simulink model "ASM_Traffic_V2X_Complete_Model_2"  (R2019a)
settings: Solver=ode1  StartTime=SIM.tstart.v  StopTime=Inf  FixedStep=SIM.StepSize.v  RelTol=1e-3
PostLoadFcn:
  | if any(exist('dsrtsu_mdlpostloadfcn', 'file') ~= 0), dsrtsu_mdlpostloadfcn('Execute', bdroot); end
  | try, asm_mdl_postloadfcn(bdroot, 'UpdateModel', 2200); catch, disp(lasterr); end,
undefined symbols (not defined in the file): _SensorPnts_1, _SensorPnts_13, _SensorPnts_17, _SensorPnts_21, _SensorPnts_25, _SensorPnts_29, _SensorPnts_33, _SensorPnts_37, _SensorPnts_41, _SensorPnts_45, _SensorPnts_49, _SensorPnts_5, _SensorPnts_53, _SensorPnts_57, _SensorPnts_9, _to_, CPT, G5A, ITS, MDL, rad, s_to_rpm, SIM
libraries: simulink x169, ASM_VehicleDynamics_lib x126, ASM_Traffic_lib x83, ASM_Utils_lib x49, mdbs x45, ASM_Environment_lib x17, dspindex x12, dsaV2xLibraryAux x10, dsmpblib x6, dsaV2xAsn1Library x4, dsaV2xLibrary x4, ASM_BrakeHydraulics_lib x4
(part 10 of 36)

== system ASM_Traffic_V2X_Complete_Model_2/IO/V2X_Subsystem/Car_Data/Fellow_ID_3 ==
  "EGO_Car_Position " : Inport
  Input : Inport  Port=2
  Bus Creator : BusCreator  Inputs=6
  Bus Creator1 : BusCreator  Inputs=2
  Bus Selector1 : BusSelector  OutputSignals=Environment.Traffic.FellowMovement.FellowPositions.Pos_Fellows_MainPnt_CoorSys_E[x;y;z][m].Pos_x_Fellows[m],Environment.Traffic.FellowMovement.FellowPositions.Pos_Fellows_MainPnt_CoorSys_E[x;y;z][m].Pos_y_Fellows[m],Environment.Traffic.FellowMovement.FellowPositions.Pos_Fellows_MainPnt_CoorSys_E[x;y;z][m].Pos_z_Fellows[m],Environment.Traffic.FellowMovement.FellowVelocities.v_Fellows[x;y;z][km|h],Environment.Traffic.FellowMovement.FellowPositions.Angle_Fellows[x;y;z][deg].Angle_Yaw_Fellows[deg],Environment.Road.UserSignals_Customized.Const_Offset_Lat[deg],Environment.Road.UserSignals_Customized.Const_Offset_Long[deg]
  Display : Display
  Display1 : Display
  Distance_Calculation : Subsystem
  Fellow_ID : Constant  Value=3
  Fellow_ID_1_Spherical_XY2GPS : Subsystem  TreatAsAtomicUnit=on
  Heading Function : MATLAB Function  TreatAsAtomicUnit=on
  Terminator2 : Terminator
  Variable Selector{,1..3} (4 alike) : dspindex/Variable Selector  NumInputs=1  rowsOrCols=Rows  IdxMode=Variable  Elements=[1 3]  ZerOneIdxMode=One-based  errmode=Clip Index  FillMode=on  FillValues=0
  Output : Outport
  wires:
  Variable Selector3/1 -> Heading Function/1(u)  "Speed"
  Heading Function/1(y) -> Bus Creator/6  "Heading"
  Bus Selector1/5 -> Variable Selector3/1  "<Angle_Yaw_Fellows[deg]>"
  Variable Selector2/1 -> Bus Creator/5  "Speed"
  Bus Selector1/4 -> Variable Selector2/1  "<v_Fellows[x;y;z][km|h]>"
  Bus Selector1/1 -> Variable Selector/1  "<Pos_x_Fellows[m]>"
  Bus Selector1/3 -> Terminator2/1  "<Pos_z_Fellows[m]>"
  Bus Selector1/2 -> Variable Selector1/1  "<Pos_y_Fellows[m]>"
  Input/1 -> Bus Selector1/1
  Distance_Calculation/1(Distance<50m) -> Bus Creator/4  "Enable"
  "EGO_Car_Position "/1 -> Distance_Calculation/3(Egocar)
  Fellow_ID_1_Spherical_XY2GPS/2(Latitude_Veh) -> Bus Creator/2  "Latitude[deg]"
  Fellow_ID/1 -> Variable Selector/2, Variable Selector1/2, Variable Selector2/2, Variable Selector3/2, Bus Creator/3  "Fellow_ID"
  Variable Selector1/1 -> Display1/1, Distance_Calculation/1(Fellow_y), Fellow_ID_1_Spherical_XY2GPS/2(Position_y_Veh)
  Fellow_ID_1_Spherical_XY2GPS/1(Longitude_Veh) -> Bus Creator/1  "Longitude[deg]"
  Bus Creator/1 -> Output/1
  Variable Selector/1 -> Display/1, Distance_Calculation/2(Fellow_x), Fellow_ID_1_Spherical_XY2GPS/1(Position_x_Veh)
  Bus Selector1/6 -> Bus Creator1/1  "<Const_Offset_Lat[deg]>"
  Bus Selector1/7 -> Bus Creator1/2  "<Const_Offset_Long[deg]>"
  Bus Creator1/1 -> Fellow_ID_1_Spherical_XY2GPS/3(Lat_Long)

== system ASM_Traffic_V2X_Complete_Model_2/IO/V2X_Subsystem/Car_Data/Subsystem ==
  In1 : Inport
  Input : Inport  Port=2
  Input1 : Inport  Port=3
  Bus Creator : BusCreator  Inputs=5
  Bus Creator1 : BusCreator  Inputs=4
  Bus Selector : BusSelector  OutputSignals=Environment.Road.UserSignals_Customized.Const_Offset_Lat[deg],Environment.Road.UserSignals_Customized.Const_Offset_Long[deg],VehicleDynamics.VehicleMovement.Velocities.Vehicle.Linear.v_Total_Vehicle[km|h]
  Bus Selector1 : BusSelector  OutputSignals=Environment.Road.Road_ASMVeh.s_Veh_Road[m]
  Bus Selector2 : BusSelector  OutputSignals=Longitude[deg],Latitude[deg],Pos_y_Vehicle_CoorSys_E[m],Pos_x_Vehicle_CoorSys_E[m]
  Out1 : Outport
  wires:
  Bus Selector/2 -> Bus Creator1/2  "<Const_Offset_Long[deg]>"
  Bus Selector/1 -> Bus Creator1/1  "<Const_Offset_Lat[deg]>"
  In1/1 -> Bus Selector/1
  Input/1 -> Bus Selector2/1
  Bus Selector2/1 -> Bus Creator/1  "<Longitude[deg]>"
  Bus Selector2/2 -> Bus Creator/2  "<Latitude[deg]>"
  Bus Selector2/3 -> Bus Creator/3  "<Pos_y_Vehicle_CoorSys_E[m]>"
  Bus Creator/1 -> Bus Creator1/4
  Bus Creator1/1 -> Out1/1  "GenDENMData"
  Bus Selector2/4 -> Bus Creator/4  "<Pos_x_Vehicle_CoorSys_E[m]>"
  Bus Selector/3 -> Bus Creator1/3  "<v_Total_Vehicle[km|h]>"
  Input1/1 -> Bus Selector1/1
  Bus Selector1/1 -> Bus Creator/5  "<s_Veh_Road[m]>"

== system ASM_Traffic_V2X_Complete_Model_2/IO/V2X_Subsystem/Subsystem/Subsystem ==
  In1 : Inport
  Trigger : TriggerPort  VariantControl=Variant  PortDimensions=1
  Output : Outport
  wires:
  In1/1 -> Output/1

== system ASM_Traffic_V2X_Complete_Model_2/MDL/Drivetrain/External Loads/ManualLoadTorque ==
  In : Inport
  LoadTorque Switch : Switch  Criteria=u2 ~= 0  SaturateOnIntegerOverflow=on
  Sum : Sum  Inputs=|++  SaturateOnIntegerOverflow=on
  Out : Outport
  wires:
  [TAG_Drivetrain_SW_LoadTorque_Mode] -> LoadTorque Switch/2
  LoadTorque Switch/1 -> Out/1
  In/1 -> Sum/2, LoadTorque Switch/3
  [TAG_Drivetrain_Const_LoadTorque] -> Sum/1
  Sum/1 -> LoadTorque Switch/1

== system ASM_Traffic_V2X_Complete_Model_2/MDL/Drivetrain/Final_Drive_Assembly/ASMSignalCollector ==
  BusCreator : BusCreator  Inputs=13
  Clutch_4WD : Subsystem
  FinalDrive_Ratio : Subsystem
  Shaft_CF : Subsystem
  Shaft_CR : Subsystem
  Shaft_TGCL4WD : Subsystem
  Transfer_Gearbox : Subsystem
  tag scope: ASMBUS_Drivetrain_FinalDriveAssembly=global
  wires:
  [ASMBUS_Drivetrain_Clutch_4WD] -> Clutch_4WD/2(Clutch_4WD)
  [ASMBUS_Drivetrain_Transfer_Gearbox] -> Transfer_Gearbox/2(Transfer_Gearbox)
  [ASMBUS_Drivetrain_Shaft_CR] -> Shaft_CR/2(Shaft_CR)
  [ASMBUS_Drivetrain_Shaft_CF] -> Shaft_CF/2(Shaft_CF)
  [ASMBUS_Drivetrain_Shaft_TGCL4WD] -> Shaft_TGCL4WD/2(Shaft_TGCL4WD)
  [TAG_Sw_Drivetrain_Mode] -> Shaft_TGCL4WD/1(Drivetrain_Mode[1|2|3|4|5]), Shaft_CF/1(Drivetrain_Mode[1|2|3|4|5]), Shaft_CR/1(Drivetrain_Mode[1|2|3|4|5]), Transfer_Gearbox/1(Drivetrain_Mode[1|2|3|4|5]), Clutch_4WD/1(Drivetrain_Mode[1|2|3|4|5]), FinalDrive_Ratio/1(Drivetrain_Mode[1|2|3|4|5])
  FinalDrive_Ratio/1(i_FinalDrive[]) -> BusCreator/1
  Shaft_CR/1(ASMSignalBus) -> BusCreator/7
  Shaft_CF/1(ASMSignalBus) -> BusCreator/6
  BusCreator/1 -> [ASMBUS_Drivetrain_FinalDriveAssembly]  "FinalDriveAssembly"
  [ASMBUS_Drivetrain_FrontDifferential] -> BusCreator/3, FinalDrive_Ratio/3(FrontDifferential)
  [ASMBUS_Drivetrain_RearDifferential] -> BusCreator/4, FinalDrive_Ratio/4(RearDifferential)
  [ASMBUS_Drivetrain_Shaft_FL] -> BusCreator/10
  [ASMBUS_Drivetrain_Shaft_FR] -> BusCreator/11
  [ASMBUS_Drivetrain_Shaft_RL] -> BusCreator/12
  [ASMBUS_Drivetrain_Shaft_RR] -> BusCreator/13
  Shaft_TGCL4WD/1(ASMSignalBus) -> BusCreator/5
  [ASMBUS_Drivetrain_CentralDifferential] -> FinalDrive_Ratio/2(CentralDifferential), BusCreator/2
  Transfer_Gearbox/1(ASMSignalBus) -> BusCreator/8
  Clutch_4WD/1(ASMSignalBus) -> BusCreator/9

== system ASM_Traffic_V2X_Complete_Model_2/MDL/Drivetrain/Final_Drive_Assembly/Differentials ==
  Inertia_Trm[kgm2] : Inport
  Trq_Out_Trm[Nm] : Inport  Port=2
  Trq_In_FrontDiff[Nm] : Inport  Port=3
  Inertia_External_InputShaft_FrontDiff[kgm2] : Inport  Port=4
  Trq_Ext_Cage_FrontDiff[Nm] : Inport  Port=5
  Inertia_Ext_Cage_FrontDiff[kgm2] : Inport  Port=6
  Trq_In_RearDiff[Nm] : Inport  Port=7
  Inertia_External_InputShaft_RearDiff[kgm2] : Inport  Port=8
  Trq_RL_Shaft[Nm] : Inport  Port=9
  Trq_RR_Shaft[Nm] : Inport  Port=10
  Trq_CR_Shaft[Nm] : Inport  Port=11
  Trq_CF_Shaft[Nm] : Inport  Port=12
  Trq_FL_Shaft[Nm] : Inport  Port=13
  Trq_FR_Shaft[Nm] : Inport  Port=14
  Reset[0|1] : Inport  Port=15
  Bus Selector1 : BusSelector  OutputSignals=Ctrl_CentralDiff[%]
  Bus Selector2 : BusSelector  OutputSignals=Ctrl_Parking_Pawl[0|1]
  Bus Selector3 : BusSelector  OutputSignals=Ctrl_FrontDiff[%]
  Bus Selector4 : BusSelector  OutputSignals=Ctrl_RearDiff[%]
  CENTRAL_DIFFERENTIAL : ASM_VehicleDynamics_lib/Drivetrain/Differential/CENTRAL_DIFFERENTIAL  Tag=ASM_SUBCOMPONENT  Const_TrqDistribution=MDL.Drivetrain.CentralDifferential.Const_TrqDistribution  Const_i_MainReductionGear=MDL.Drivetrain.CentralDifferential.Const_i_MainReductionGear  Const_i_InnerGear=MDL.Drivetrain.CentralDifferential.Const_i_InnerGear  Const_Inertia_FrontSideGear=MDL.Drivetrain.CentralDifferential.Const_Inertia_FrontSideGear  Const_Inertia_RearSideGear=MDL.Drivetrain.CentralDifferential.Const_Inertia_RearSideGear  Const_Inertia_InnerGear=MDL.Drivetrain.CentralDifferential.Const_Inertia_InnerGear  Const_Inertia_MainReductionGear=MDL.Drivetrain.CentralDifferential.Const_Inertia_MainReductionGear  Const_Inertia_InputGear=MDL.Drivetrain.CentralDifferential.Const_Inertia_InputGear  Sw_DifferentialLock_Mode=MDL.Drivetrain.CentralDifferential.Sw_DifferentialLock_Mode  Const_Trq_Max_LockClutch=MDL.Drivetrain.CentralDifferential.Const_Trq_Max_LockClutch  Const_Coef_DynamicClutchTrq=MDL.Drivetrain.CentralDifferential.Const_Coef_DynamicClutchTrq  Const_Ctrl_Offset_LockClutch=MDL.Drivetrain.CentralDifferential.Const_Ctrl_Offset_LockClutch  StepSize=SIM.StepSize  ASMProperties=struct('Name','CENTRAL_DIFFERENTIAL','Version','8.0','Library','ASM_VehicleDynamics_lib')  ASMInstanceName=central_differential  ASMInstanceID=1
  Ctrl_Parking_Pawl_FrontDiff[0|1] : Constant  Value=0
  Ctrl_Parking_Pawl_RearDiff[0|1] : Constant  Value=0
  FROM_STABILIZATION_CENTRAL_DIFFERENTIAL : ASM_VehicleDynamics_lib/Drivetrain/Stabilization/FROM_STABILIZATION  Tag=ASM_SUBCOMPONENT  Stabi_Block=CENTRAL_DIFFERENTIAL  Stabi_Block_ID=1  ASMProperties=struct('Name','FROM_STABILIZATION','Version','1.0','Library','ASM_VehicleDynamics_lib')  ASMInstanceName=from_stabilization  ASMInstanceID=1
      settings: AttributesFormatString=Destination: CENTRAL_DIFFERENTIAL_ID1
  FROM_STABILIZATION_FRONT_DIFFERENTIAL : ASM_VehicleDynamics_lib/Drivetrain/Stabilization/FROM_STABILIZATION  Tag=ASM_SUBCOMPONENT  Stabi_Block=FRONT_DIFFERENTIAL  Stabi_Block_ID=1  ASMProperties=struct('Name','FROM_STABILIZATION','Version','1.0','Library','ASM_VehicleDynamics_lib')  ASMInstanceName=from_stabilization  ASMInstanceID=1
      settings: AttributesFormatString=Destination: FRONT_DIFFERENTIAL_ID1
  FROM_STABILIZATION_REAR_DIFFERENTIAL : ASM_VehicleDynamics_lib/Drivetrain/Stabilization/FROM_STABILIZATION  Tag=ASM_SUBCOMPONENT  Stabi_Block=REAR_DIFFERENTIAL  Stabi_Block_ID=1  ASMProperties=struct('Name','FROM_STABILIZATION','Version','1.0','Library','ASM_VehicleDynamics_lib')  ASMInstanceName=from_stabilization  ASMInstanceID=1
      settings: AttributesFormatString=Destination: REAR_DIFFERENTIAL_ID1
  FRONT_DIFFERENTIAL : ASM_VehicleDynamics_lib/Drivetrain/Differential/FRONT_DIFFERENTIAL  Tag=ASM_SUBCOMPONENT  Const_i_MainReductionGear=MDL.Drivetrain.FrontDifferential.Const_i_MainReductionGear  Const_i_InnerGear=MDL.Drivetrain.FrontDifferential.Const_i_InnerGear  Const_Inertia_LeftSideGear=MDL.Drivetrain.FrontDifferential.Const_Inertia_LeftSideGear  Const_Inertia_RightSideGear=MDL.Drivetrain.FrontDifferential.Const_Inertia_RightSideGear  Const_Inertia_InnerGear=MDL.Drivetrain.FrontDifferential.Const_Inertia_InnerGear  Const_Inertia_MainReductionGear=MDL.Drivetrain.FrontDifferential.Const_Inertia_MainReductionGear  Const_Inertia_InputGear=MDL.Drivetrain.FrontDifferential.Const_Inertia_InputGear  Sw_DifferentialLock_Mode=MDL.Drivetrain.FrontDifferential.Sw_DifferentialLock_Mode  Const_Trq_Max_LockClutch=MDL.Drivetrain.FrontDifferential.Const_Trq_Max_LockClutch  Const_Coef_DynamicClutchTrq=MDL.Drivetrain.FrontDifferential.Const_Coef_DynamicClutchTrq  Const_Ctrl_Offset_LockClutch=MDL.Drivetrain.FrontDifferential.Const_Ctrl_Offset_LockClutch  StepSize=SIM.StepSize  ASMProperties=struct('Name','FRONT_DIFFERENTIAL','Version','8.0','Library','ASM_VehicleDynamics_lib')  ASMInstanceName=front_differential  ASMInstanceID=1
  Inertia_Ext_Cage_CentralDiff[kgm2] : Constant  Value=0
  Inertia_Ext_Cage_RearDiff[kgm2] : Constant  Value=0
  REAR_DIFFERENTIAL : ASM_VehicleDynamics_lib/Drivetrain/Differential/REAR_DIFFERENTIAL  Tag=ASM_SUBCOMPONENT  Const_i_MainReductionGear=MDL.Drivetrain.RearDifferential.Const_i_MainReductionGear  Const_i_InnerGear=MDL.Drivetrain.RearDifferential.Const_i_InnerGear  Const_Inertia_LeftSideGear=MDL.Drivetrain.RearDifferential.Const_Inertia_LeftSideGear  Const_Inertia_RightSideGear=MDL.Drivetrain.RearDifferential.Const_Inertia_RightSideGear  Const_Inertia_InnerGear=MDL.Drivetrain.RearDifferential.Const_Inertia_InnerGear  Const_Inertia_MainReductionGear=MDL.Drivetrain.RearDifferential.Const_Inertia_MainReductionGear  Const_Inertia_InputGear=MDL.Drivetrain.RearDifferential.Const_Inertia_InputGear  Sw_DifferentialLock_Mode=MDL.Drivetrain.RearDifferential.Sw_DifferentialLock_Mode  Const_Trq_Max_LockClutch=MDL.Drivetrain.RearDifferential.Const_Trq_Max_LockClutch  Const_Coef_DynamicClutchTrq=MDL.Drivetrain.RearDifferential.Const_Coef_DynamicClutchTrq  Const_Ctrl_Offset_LockClutch=MDL.Drivetrain.RearDifferential.Const_Ctrl_Offset_LockClutch  StepSize=SIM.StepSize  ASMProperties=struct('Name','REAR_DIFFERENTIAL','Version','8.0','Library','ASM_VehicleDynamics_lib')  ASMInstanceName=rear_differential  ASMInstanceID=1
  Saturation[1_3] : Saturate  UpperLimit=3  LowerLimit=1
  SignalSelection : Subsystem
  TO_STABILIZATION_CENTRAL_DIFFERENTIAL : ASM_VehicleDynamics_lib/Drivetrain/Stabilization/TO_STABILIZATION  Tag=ASM_SUBCOMPONENT  Stabi_Block=CENTRAL_DIFFERENTIAL  Stabi_Block_ID=1  ASMProperties=struct('Name','TO_STABILIZATION','Version','1.0','Library','ASM_VehicleDynamics_lib')  ASMInstanceName=to_stabilization  ASMInstanceID=1
      settings: AttributesFormatString=Source: CENTRAL_DIFFERENTIAL_ID1
  TO_STABILIZATION_FRONT_DIFFERENTIAL : ASM_VehicleDynamics_lib/Drivetrain/Stabilization/TO_STABILIZATION  Tag=ASM_SUBCOMPONENT  Stabi_Block=FRONT_DIFFERENTIAL  Stabi_Block_ID=1  ASMProperties=struct('Name','TO_STABILIZATION','Version','1.0','Library','ASM_VehicleDynamics_lib')  ASMInstanceName=to_stabilization  ASMInstanceID=1
      settings: AttributesFormatString=Source: FRONT_DIFFERENTIAL_ID1
  TO_STABILIZATION_REAR_DIFFERENTIAL : ASM_VehicleDynamics_lib/Drivetrain/Stabilization/TO_STABILIZATION  Tag=ASM_SUBCOMPONENT  Stabi_Block=REAR_DIFFERENTIAL  Stabi_Block_ID=1  ASMProperties=struct('Name','TO_STABILIZATION','Version','1.0','Library','ASM_VehicleDynamics_lib')  ASMInstanceName=to_stabilization  ASMInstanceID=1
      settings: AttributesFormatString=Source: REAR_DIFFERENTIAL_ID1
  Trq_Ext_Cage_CentralDiff[Nm] : Constant  Value=0
  Trq_Ext_Cage_RearDiff[Nm] : Constant  Value=0
  omega_Cage_CentralDiff[rad|s] : Terminator
  omega_Cage_RearDiff[rad|s] : Terminator
  omega_Out_Front_Init_CentralDiff[rad|s] : Constant  Value=0
  omega_Out_Left_Init_FrontDiff[rad|s] : Constant  Value=0
  omega_Out_Left_Init_RearDiff[rad|s] : Constant  Value=0
  omega_Out_Rear_Init_CentralDiff[rad|s] : Constant  Value=0
  omega_Out_Right_Init_FrontDiff[rad|s] : Constant  Value=0
  omega_Out_Right_Init_RearDiff[rad|s] : Constant  Value=0
  omega_In_Diff[rad|s] : Outport
  omega_Cage_FrontDiff[rad|s] : Outport  Port=2
  omega_In_RearDiff[rad|s] : Outport  Port=3
  omega_In_FrontDiff[rad|s] : Outport  Port=4
  omega_Out_Front_CentralDiff[rad|s] : Outport  Port=5
  omega_Out_Rear_CentralDiff[rad|s] : Outport  Port=6
  omega_Out_Left_FrontDiff[rad|s] : Outport  Port=7
  omega_Out_Right_FrontDiff[rad|s] : Outport  Port=8
  omega_Out_Left_RearDiff[rad|s] : Outport  Port=9
  omega_Out_Right_RearDiff[rad|s] : Outport  Port=10
  tag scope: ASMBUS_Drivetrain_CentralDifferential=scoped, ASMBUS_Drivetrain_FrontDifferential=scoped, ASMBUS_Drivetrain_RearDifferential=scoped
  wires:
  omega_Out_Right_Init_RearDiff[rad|s]/1 -> REAR_DIFFERENTIAL/11
  Trq_Ext_Cage_RearDiff[Nm]/1 -> REAR_DIFFERENTIAL/7
  omega_Out_Left_Init_RearDiff[rad|s]/1 -> REAR_DIFFERENTIAL/10
  Inertia_Ext_Cage_RearDiff[kgm2]/1 -> REAR_DIFFERENTIAL/8
  Ctrl_Parking_Pawl_RearDiff[0|1]/1 -> REAR_DIFFERENTIAL/9
  REAR_DIFFERENTIAL/5 -> omega_Cage_RearDiff[rad|s]/1
  omega_Out_Right_Init_FrontDiff[rad|s]/1 -> FRONT_DIFFERENTIAL/11
  omega_Out_Left_Init_FrontDiff[rad|s]/1 -> FRONT_DIFFERENTIAL/10
  Ctrl_Parking_Pawl_FrontDiff[0|1]/1 -> FRONT_DIFFERENTIAL/9
  FRONT_DIFFERENTIAL/1 -> [ASMBUS_Drivetrain_FrontDifferential]
  Inertia_Ext_Cage_CentralDiff[kgm2]/1 -> CENTRAL_DIFFERENTIAL/10
  Trq_Ext_Cage_CentralDiff[Nm]/1 -> CENTRAL_DIFFERENTIAL/9
  omega_Out_Front_Init_CentralDiff[rad|s]/1 -> CENTRAL_DIFFERENTIAL/11
  omega_Out_Rear_Init_CentralDiff[rad|s]/1 -> CENTRAL_DIFFERENTIAL/12
  CENTRAL_DIFFERENTIAL/5 -> omega_Cage_CentralDiff[rad|s]/1
  CENTRAL_DIFFERENTIAL/4 -> omega_Out_Rear_CentralDiff[rad|s]/1
  CENTRAL_DIFFERENTIAL/3 -> omega_Out_Front_CentralDiff[rad|s]/1
  CENTRAL_DIFFERENTIAL/2 -> SignalSelection/1(omega_In_CentralDiff[rad|s])
  CENTRAL_DIFFERENTIAL/1 -> [ASMBUS_Drivetrain_CentralDifferential]
  Reset[0|1]/1 -> CENTRAL_DIFFERENTIAL/7, REAR_DIFFERENTIAL/5, FRONT_DIFFERENTIAL/5
  Saturation[1_3]/1 -> CENTRAL_DIFFERENTIAL/4
  [TAG_Sw_Drivetrain_Mode] -> Saturation[1_3]/1
  SignalSelection/1(omega_In_Diff[rad|s]) -> omega_In_Diff[rad|s]/1
  Inertia_Ext_Cage_FrontDiff[kgm2]/1 -> FRONT_DIFFERENTIAL/8
  Trq_Ext_Cage_FrontDiff[Nm]/1 -> FRONT_DIFFERENTIAL/7
  Trq_In_RearDiff[Nm]/1 -> REAR_DIFFERENTIAL/1
  Trq_CF_Shaft[Nm]/1 -> CENTRAL_DIFFERENTIAL/6
  REAR_DIFFERENTIAL/2 -> omega_In_RearDiff[rad|s]/1
  FRONT_DIFFERENTIAL/2 -> SignalSelection/2(omega_In_FrontDiff[rad|s]), omega_In_FrontDiff[rad|s]/1
  [TAG_FromIO_Drivetrain] -> Bus Selector1/1, Bus Selector2/1, Bus Selector3/1, Bus Selector4/1
  Trq_In_FrontDiff[Nm]/1 -> FRONT_DIFFERENTIAL/1
  Bus Selector1/1 -> CENTRAL_DIFFERENTIAL/3  "<Ctrl_CentralDiff[%]>"
  Bus Selector3/1 -> FRONT_DIFFERENTIAL/2  "<Ctrl_FrontDiff[%]>"
  Trq_CR_Shaft[Nm]/1 -> CENTRAL_DIFFERENTIAL/5
  FRONT_DIFFERENTIAL/5 -> omega_Cage_FrontDiff[rad|s]/1
  Inertia_External_InputShaft_FrontDiff[kgm2]/1 -> FRONT_DIFFERENTIAL/6
  Bus Selector4/1 -> REAR_DIFFERENTIAL/2  "<Ctrl_RearDiff[%]>"
  Inertia_Trm[kgm2]/1 -> CENTRAL_DIFFERENTIAL/1
  Trq_Out_Trm[Nm]/1 -> CENTRAL_DIFFERENTIAL/2
  REAR_DIFFERENTIAL/1 -> [ASMBUS_Drivetrain_RearDifferential]
  Inertia_External_InputShaft_RearDiff[kgm2]/1 -> REAR_DIFFERENTIAL/6
  Bus Selector2/1 -> CENTRAL_DIFFERENTIAL/8  "<Ctrl_Parking_Pawl[0|1]>"
  Trq_RL_Shaft[Nm]/1 -> REAR_DIFFERENTIAL/3
  Trq_RR_Shaft[Nm]/1 -> REAR_DIFFERENTIAL/4
  REAR_DIFFERENTIAL/3 -> omega_Out_Left_RearDiff[rad|s]/1
  Trq_FR_Shaft[Nm]/1 -> FRONT_DIFFERENTIAL/4
  REAR_DIFFERENTIAL/4 -> omega_Out_Right_RearDiff[rad|s]/1
  FRONT_DIFFERENTIAL/3 -> omega_Out_Left_FrontDiff[rad|s]/1
  FRONT_DIFFERENTIAL/4 -> omega_Out_Right_FrontDiff[rad|s]/1
  Trq_FL_Shaft[Nm]/1 -> FRONT_DIFFERENTIAL/3
  FRONT_DIFFERENTIAL/6 -> TO_STABILIZATION_FRONT_DIFFERENTIAL/1
  REAR_DIFFERENTIAL/6 -> TO_STABILIZATION_REAR_DIFFERENTIAL/1
  FROM_STABILIZATION_REAR_DIFFERENTIAL/1 -> REAR_DIFFERENTIAL/12
  FROM_STABILIZATION_FRONT_DIFFERENTIAL/1 -> FRONT_DIFFERENTIAL/12
  CENTRAL_DIFFERENTIAL/6 -> TO_STABILIZATION_CENTRAL_DIFFERENTIAL/1
  FROM_STABILIZATION_CENTRAL_DIFFERENTIAL/1 -> CENTRAL_DIFFERENTIAL/13

== system ASM_Traffic_V2X_Complete_Model_2/MDL/Drivetrain/Final_Drive_Assembly/FF4WD_Parts ==
  Trq_RL_Shaft[Nm] : Inport
  Trq_RR_Shaft[Nm] : Inport  Port=2
  Reset[0|1] : Inport  Port=3
  omega_In_RearDiff[rad|s] : Inport  Port=4
  omega_Cage_FrontDiff[rad|s] : Inport  Port=5
  Bus Selector1 : BusSelector  OutputSignals=Const_i_MainReductionGear[]
  Bus Selector4 : BusSelector  OutputSignals=Ctrl_Clutch_4WD[%]
  CLUTCH_4WD : ASM_VehicleDynamics_lib/Drivetrain/Clutch/CLUTCH_4WD  Tag=ASM_SUBCOMPONENT  Const_Inertia_InputSide=MDL.Drivetrain.Clutch_4WD.Const_Inertia_InputSide  Const_Inertia_OutputSide=MDL.Drivetrain.Clutch_4WD.Const_Inertia_OutputSide  Const_Torque_Max=MDL.Drivetrain.Clutch_4WD.Const_Torque_Max  Map_Trq_Clutch_Red=MDL.Drivetrain.Clutch_4WD.Map_Trq_Clutch_Red  Const_Coef_DynamicClutchTrq=MDL.Drivetrain.Clutch_4WD.Const_Coef_DynamicClutchTrq  StepSize=SIM.StepSize  ASMProperties=struct('Name','CLUTCH_4WD','Version','6.0','Library','ASM_VehicleDynamics_lib')  ASMInstanceName=clutch_4wd  ASMInstanceID=1
  FROM_STABILIZATION_CLUTCH_4WD : ASM_VehicleDynamics_lib/Drivetrain/Stabilization/FROM_STABILIZATION  Tag=ASM_SUBCOMPONENT  Stabi_Block=CLUTCH_4WD  Stabi_Block_ID=1  ASMProperties=struct('Name','FROM_STABILIZATION','Version','1.0','Library','ASM_VehicleDynamics_lib')  ASMInstanceName=from_stabilization  ASMInstanceID=1
      settings: AttributesFormatString=Destination: CLUTCH_4WD_ID1
  Map_Mode_2_Parameter : Lookup_n-D  NumberOfTableDimensions=1  BreakpointsForDimension1=[1:5]  Table=[1 2 3 1 2]  InternalRulePriority=Speed  RndMeth=Simplest  InputSameDT=on
      settings: AttributesFormatString=Map FF => FWD & FF4WD => AWD
  SHAFT_TGCL4WD : ASM_VehicleDynamics_lib/Drivetrain/Shaft/SHAFT_TGCL4WD  Tag=ASM_SUBCOMPONENT  Const_Stiffness_Shaft_TGCL4WD=MDL.Drivetrain.Shaft_TGCL4WD.Const_Stiffness  Const_Damping_Shaft_TGCL4WD=MDL.Drivetrain.Shaft_TGCL4WD.Const_Damping  StepSize=SIM.StepSize  ASMProperties=struct('Name','SHAFT_TGCL4WD','Version','4.0','Library','ASM_VehicleDynamics_lib')  ASMInstanceName=Shafts  ASMInstanceID=1
  TO_STABILIZATION_CLUTCH_4WD : ASM_VehicleDynamics_lib/Drivetrain/Stabilization/TO_STABILIZATION  Tag=ASM_SUBCOMPONENT  Stabi_Block=CLUTCH_4WD  Stabi_Block_ID=1  ASMProperties=struct('Name','TO_STABILIZATION','Version','1.0','Library','ASM_VehicleDynamics_lib')  ASMInstanceName=to_stabilization  ASMInstanceID=1
      settings: AttributesFormatString=Source: CLUTCH_4WD_ID1
  TO_STABILIZATION_SHAFT_TGCL4WD : ASM_VehicleDynamics_lib/Drivetrain/Stabilization/TO_STABILIZATION  Tag=ASM_SUBCOMPONENT  Stabi_Block=SHAFT_TGCL4WD  Stabi_Block_ID=1  ASMProperties=struct('Name','TO_STABILIZATION','Version','1.0','Library','ASM_VehicleDynamics_lib')  ASMInstanceName=to_stabilization  ASMInstanceID=1
      settings: AttributesFormatString=Source: SHAFT_TGCL4WD_ID1
  TO_STABILIZATION_TRANSFER_GEARBOX : ASM_VehicleDynamics_lib/Drivetrain/Stabilization/TO_STABILIZATION  Tag=ASM_SUBCOMPONENT  Stabi_Block=TRANSFER_GEARBOX  Stabi_Block_ID=1  ASMProperties=struct('Name','TO_STABILIZATION','Version','1.0','Library','ASM_VehicleDynamics_lib')  ASMInstanceName=to_stabilization  ASMInstanceID=1
      settings: AttributesFormatString=Source: TRANSFER_GEARBOX_ID1
  TRANSFER_GEARBOX : ASM_VehicleDynamics_lib/Drivetrain/Gearbox/TRANSFER_GEARBOX  Tag=ASM_SUBCOMPONENT  Const_GearRatio=MDL.Drivetrain.TransferGearbox.Const_GearRatio  Const_Inertia_Output_Gear=MDL.Drivetrain.TransferGearbox.Const_Inertia_Output_Gear  Const_Inertia_Input_Gear=MDL.Drivetrain.TransferGearbox.Const_Inertia_Input_Gear  ASMProperties=struct('Name','TRANSFER_GEARBOX','Version','4.0','Library','ASM_VehicleDynamics_lib')  ASMInstanceName=transfer_gearbox  ASMInstanceID=1
  omega_Clutch_4WD_In_Init[rad|s] : Constant  Value=0
  Inertia_Out_Clutch4WD[kgm2] : Outport
  Trq_Lock_Clutch4WD[Nm] : Outport  Port=2
  Inertia_In_TransferGearbox[kgm2] : Outport  Port=3
  Trq_In_TransferGearbox[Nm] : Outport  Port=4
  tag scope: ASMBUS_Drivetrain_Clutch_4WD=scoped, ASMBUS_Drivetrain_Shaft_TGCL4WD=scoped, ASMBUS_Drivetrain_Transfer_Gearbox=scoped
  wires:
  omega_Cage_FrontDiff[rad|s]/1 -> TRANSFER_GEARBOX/3
  omega_Clutch_4WD_In_Init[rad|s]/1 -> CLUTCH_4WD/8
  Bus Selector1/1 -> CLUTCH_4WD/7  "<Const_i_MainReductionGear[]>"
  [ASMBUS_Drivetrain_RearDifferential] -> Bus Selector1/1
  TRANSFER_GEARBOX/3 -> Inertia_In_TransferGearbox[kgm2]/1
  TRANSFER_GEARBOX/2 -> Trq_In_TransferGearbox[Nm]/1
  TRANSFER_GEARBOX/1 -> [ASMBUS_Drivetrain_Transfer_Gearbox]
  CLUTCH_4WD/4 -> Inertia_Out_Clutch4WD[kgm2]/1
  CLUTCH_4WD/3 -> Trq_Lock_Clutch4WD[Nm]/1
  SHAFT_TGCL4WD/1 -> [ASMBUS_Drivetrain_Shaft_TGCL4WD]
  [TAG_FromIO_Drivetrain] -> Bus Selector4/1
  Bus Selector4/1 -> CLUTCH_4WD/2  "<Ctrl_Clutch_4WD[%]>"
  [TAG_Sw_Drivetrain_Mode] -> Map_Mode_2_Parameter/1
  Map_Mode_2_Parameter/1 -> SHAFT_TGCL4WD/3, TRANSFER_GEARBOX/1
  Reset[0|1]/1 -> CLUTCH_4WD/6, SHAFT_TGCL4WD/4
  omega_In_RearDiff[rad|s]/1 -> CLUTCH_4WD/5
  Trq_RR_Shaft[Nm]/1 -> CLUTCH_4WD/4
  Trq_RL_Shaft[Nm]/1 -> CLUTCH_4WD/3
  CLUTCH_4WD/2 -> SHAFT_TGCL4WD/2
  TRANSFER_GEARBOX/4 -> SHAFT_TGCL4WD/1
  SHAFT_TGCL4WD/2 -> CLUTCH_4WD/1, TRANSFER_GEARBOX/2
  CLUTCH_4WD/1 -> [ASMBUS_Drivetrain_Clutch_4WD]
  TRANSFER_GEARBOX/5 -> TO_STABILIZATION_TRANSFER_GEARBOX/1
  SHAFT_TGCL4WD/3 -> TO_STABILIZATION_SHAFT_TGCL4WD/1
  CLUTCH_4WD/5 -> TO_STABILIZATION_CLUTCH_4WD/1
  FROM_STABILIZATION_CLUTCH_4WD/1 -> CLUTCH_4WD/9

== system ASM_Traffic_V2X_Complete_Model_2/MDL/Drivetrain/Final_Drive_Assembly/STABILIZATION ==
  DRIVETRAIN_STABILIZATION : ASM_VehicleDynamics_lib/Drivetrain/Stabilization/DRIVETRAIN_STABILIZATION  Tag=ASM_SUBCOMPONENT  StepSize=SIM.StepSize  ASMProperties=struct('Name','DRIVETRAIN_STABILIZATION','Version','1.0','Library','ASM_VehicleDynamics_lib')  ASMInstanceName=drivetrain_stabilization  ASMInstanceID=1
  FROM_ASM_CENTRAL_DIFFERENTIAL : ASM_VehicleDynamics_lib/Drivetrain/Stabilization/FROM_ASM  Tag=ASM_SUBCOMPONENT  Stabi_Block=CENTRAL_DIFFERENTIAL  Stabi_Block_ID=1  ASMProperties=struct('Name','FROM_ASM','Version','1.0','Library','ASM_VehicleDynamics_lib')  ASMInstanceName=from_asm  ASMInstanceID=1
      settings: AttributesFormatString=Source: CENTRAL_DIFFERENTIAL_ID1
  FROM_ASM_CLUTCH : ASM_VehicleDynamics_lib/Drivetrain/Stabilization/FROM_ASM  Tag=ASM_SUBCOMPONENT  Stabi_Block=CLUTCH  Stabi_Block_ID=1  ASMProperties=struct('Name','FROM_ASM','Version','1.0','Library','ASM_VehicleDynamics_lib')  ASMInstanceName=from_asm  ASMInstanceID=1
      settings: AttributesFormatString=Source: CLUTCH_ID1
  FROM_ASM_CLUTCH_4WD : ASM_VehicleDynamics_lib/Drivetrain/Stabilization/FROM_ASM  Tag=ASM_SUBCOMPONENT  Stabi_Block=CLUTCH_4WD  Stabi_Block_ID=1  ASMProperties=struct('Name','FROM_ASM','Version','1.0','Library','ASM_VehicleDynamics_lib')  ASMInstanceName=from_asm  ASMInstanceID=1
      settings: AttributesFormatString=Source: CLUTCH_4WD_ID1
  FROM_ASM_CRANK_SHAFT : ASM_VehicleDynamics_lib/Drivetrain/Stabilization/FROM_ASM  Tag=ASM_SUBCOMPONENT  Stabi_Block=CRANK_SHAFT  Stabi_Block_ID=1  ASMProperties=struct('Name','FROM_ASM','Version','1.0','Library','ASM_VehicleDynamics_lib')  ASMInstanceName=from_asm  ASMInstanceID=1
      settings: AttributesFormatString=Source: CRANK_SHAFT_ID1
  FROM_ASM_FRONT_DIFFERENTIAL : ASM_VehicleDynamics_lib/Drivetrain/Stabilization/FROM_ASM  Tag=ASM_SUBCOMPONENT  Stabi_Block=FRONT_DIFFERENTIAL  Stabi_Block_ID=1  ASMProperties=struct('Name','FROM_ASM','Version','1.0','Library','ASM_VehicleDynamics_lib')  ASMInstanceName=from_asm  ASMInstanceID=1
      settings: AttributesFormatString=Source: FRONT_DIFFERENTIAL_ID1
  FROM_ASM_GEARBOX : ASM_VehicleDynamics_lib/Drivetrain/Stabilization/FROM_ASM  Tag=ASM_SUBCOMPONENT  Stabi_Block=GEARBOX  Stabi_Block_ID=1  ASMProperties=struct('Name','FROM_ASM','Version','1.0','Library','ASM_VehicleDynamics_lib')  ASMInstanceName=from_asm  ASMInstanceID=1
      settings: AttributesFormatString=Source: GEARBOX_ID1
  FROM_ASM_REAR_DIFFERENTIAL : ASM_VehicleDynamics_lib/Drivetrain/Stabilization/FROM_ASM  Tag=ASM_SUBCOMPONENT  Stabi_Block=REAR_DIFFERENTIAL  Stabi_Block_ID=1  ASMProperties=struct('Name','FROM_ASM','Version','1.0','Library','ASM_VehicleDynamics_lib')  ASMInstanceName=from_asm  ASMInstanceID=1
      settings: AttributesFormatString=Source: REAR_DIFFERENTIAL_ID1
  FROM_ASM_SHAFT_CF : ASM_VehicleDynamics_lib/Drivetrain/Stabilization/FROM_ASM  Tag=ASM_SUBCOMPONENT  Stabi_Block=SHAFT_CF  Stabi_Block_ID=1  ASMProperties=struct('Name','FROM_ASM','Version','1.0','Library','ASM_VehicleDynamics_lib')  ASMInstanceName=from_asm  ASMInstanceID=1
      settings: AttributesFormatString=Source: SHAFT_CF_ID1
  FROM_ASM_SHAFT_CR : ASM_VehicleDynamics_lib/Drivetrain/Stabilization/FROM_ASM  Tag=ASM_SUBCOMPONENT  Stabi_Block=SHAFT_CR  Stabi_Block_ID=1  ASMProperties=struct('Name','FROM_ASM','Version','1.0','Library','ASM_VehicleDynamics_lib')  ASMInstanceName=from_asm  ASMInstanceID=1
      settings: AttributesFormatString=Source: SHAFT_CR_ID1
  FROM_ASM_SHAFT_FL : ASM_VehicleDynamics_lib/Drivetrain/Stabilization/FROM_ASM  Tag=ASM_SUBCOMPONENT  Stabi_Block=SHAFT_FL  Stabi_Block_ID=1  ASMProperties=struct('Name','FROM_ASM','Version','1.0','Library','ASM_VehicleDynamics_lib')  ASMInstanceName=from_asm  ASMInstanceID=1
      settings: AttributesFormatString=Source: SHAFT_FL_ID1
  FROM_ASM_SHAFT_FR : ASM_VehicleDynamics_lib/Drivetrain/Stabilization/FROM_ASM  Tag=ASM_SUBCOMPONENT  Stabi_Block=SHAFT_FR  Stabi_Block_ID=1  ASMProperties=struct('Name','FROM_ASM','Version','1.0','Library','ASM_VehicleDynamics_lib')  ASMInstanceName=from_asm  ASMInstanceID=1
      settings: AttributesFormatString=Source: SHAFT_FR_ID1
  FROM_ASM_SHAFT_RL : ASM_VehicleDynamics_lib/Drivetrain/Stabilization/FROM_ASM  Tag=ASM_SUBCOMPONENT  Stabi_Block=SHAFT_RL  Stabi_Block_ID=1  ASMProperties=struct('Name','FROM_ASM','Version','1.0','Library','ASM_VehicleDynamics_lib')  ASMInstanceName=from_asm  ASMInstanceID=1
      settings: AttributesFormatString=Source: SHAFT_RL_ID1
  FROM_ASM_SHAFT_RR : ASM_VehicleDynamics_lib/Drivetrain/Stabilization/FROM_ASM  Tag=ASM_SUBCOMPONENT  Stabi_Block=SHAFT_RR  Stabi_Block_ID=1  ASMProperties=struct('Name','FROM_ASM','Version','1.0','Library','ASM_VehicleDynamics_lib')  ASMInstanceName=from_asm  ASMInstanceID=1
      settings: AttributesFormatString=Source: SHAFT_RR_ID1
  FROM_ASM_SHAFT_TGCL4WD : ASM_VehicleDynamics_lib/Drivetrain/Stabilization/FROM_ASM  Tag=ASM_SUBCOMPONENT  Stabi_Block=SHAFT_TGCL4WD  Stabi_Block_ID=1  ASMProperties=struct('Name','FROM_ASM','Version','1.0','Library','ASM_VehicleDynamics_lib')  ASMInstanceName=from_asm  ASMInstanceID=1
      settings: AttributesFormatString=Source: SHAFT_TGCL4WD_ID1
  FROM_ASM_TORQUE_CONVERTER : ASM_VehicleDynamics_lib/Drivetrain/Stabilization/FROM_ASM  Tag=ASM_SUBCOMPONENT  Stabi_Block=TORQUE_CONVERTER  Stabi_Block_ID=1  ASMProperties=struct('Name','FROM_ASM','Version','1.0','Library','ASM_VehicleDynamics_lib')  ASMInstanceName=from_asm  ASMInstanceID=1
      settings: AttributesFormatString=Source: TORQUE_CONVERTER_ID1
  FROM_ASM_TRANSFER_GEARBOX : ASM_VehicleDynamics_lib/Drivetrain/Stabilization/FROM_ASM  Tag=ASM_SUBCOMPONENT  Stabi_Block=TRANSFER_GEARBOX  Stabi_Block_ID=1  ASMProperties=struct('Name','FROM_ASM','Version','1.0','Library','ASM_VehicleDynamics_lib')  ASMInstanceName=from_asm  ASMInstanceID=1
      settings: AttributesFormatString=Source: TRANSFER_GEARBOX_ID1
  Saturation[1_5] : Saturate  UpperLimit=5  LowerLimit=1
  TO_ASM_CENTRAL_DIFFERENTIAL : ASM_VehicleDynamics_lib/Drivetrain/Stabilization/TO_ASM  Tag=ASM_SUBCOMPONENT  Stabi_Block=CENTRAL_DIFFERENTIAL  Stabi_Block_ID=1  ASMProperties=struct('Name','TO_ASM','Version','1.0','Library','ASM_VehicleDynamics_lib')  ASMInstanceName=to_asm  ASMInstanceID=1
      settings: AttributesFormatString=Destination: CENTRAL_DIFFERENTIAL_ID1
  TO_ASM_CLUTCH : ASM_VehicleDynamics_lib/Drivetrain/Stabilization/TO_ASM  Tag=ASM_SUBCOMPONENT  Stabi_Block=CLUTCH  Stabi_Block_ID=1  ASMProperties=struct('Name','TO_ASM','Version','1.0','Library','ASM_VehicleDynamics_lib')  ASMInstanceName=to_asm  ASMInstanceID=1
      settings: AttributesFormatString=Destination: CLUTCH_ID1
  TO_ASM_CLUTCH_4WD : ASM_VehicleDynamics_lib/Drivetrain/Stabilization/TO_ASM  Tag=ASM_SUBCOMPONENT  Stabi_Block=CLUTCH_4WD  Stabi_Block_ID=1  ASMProperties=struct('Name','TO_ASM','Version','1.0','Library','ASM_VehicleDynamics_lib')  ASMInstanceName=to_asm  ASMInstanceID=1
      settings: AttributesFormatString=Destination: CLUTCH_4WD_ID1
  TO_ASM_CRANK_SHAFT : ASM_VehicleDynamics_lib/Drivetrain/Stabilization/TO_ASM  Tag=ASM_SUBCOMPONENT  Stabi_Block=CRANK_SHAFT  Stabi_Block_ID=1  ASMProperties=struct('Name','TO_ASM','Version','1.0','Library','ASM_VehicleDynamics_lib')  ASMInstanceName=to_asm  ASMInstanceID=1
      settings: AttributesFormatString=Destination: CRANK_SHAFT_ID1
  TO_ASM_FRONT_DIFFERENTIAL : ASM_VehicleDynamics_lib/Drivetrain/Stabilization/TO_ASM  Tag=ASM_SUBCOMPONENT  Stabi_Block=FRONT_DIFFERENTIAL  Stabi_Block_ID=1  ASMProperties=struct('Name','TO_ASM','Version','1.0','Library','ASM_VehicleDynamics_lib')  ASMInstanceName=to_asm  ASMInstanceID=1
      settings: AttributesFormatString=Destination: FRONT_DIFFERENTIAL_ID1
  TO_ASM_REAR_DIFFERENTIAL : ASM_VehicleDynamics_lib/Drivetrain/Stabilization/TO_ASM  Tag=ASM_SUBCOMPONENT  Stabi_Block=REAR_DIFFERENTIAL  Stabi_Block_ID=1  ASMProperties=struct('Name','TO_ASM','Version','1.0','Library','ASM_VehicleDynamics_lib')  ASMInstanceName=to_asm  ASMInstanceID=1
      settings: AttributesFormatString=Destination: REAR_DIFFERENTIAL_ID1
  wires:
  [TAG_Sw_Drivetrain_Mode] -> Saturation[1_5]/1
  Saturation[1_5]/1 -> DRIVETRAIN_STABILIZATION/1
  DRIVETRAIN_STABILIZATION/1 -> TO_ASM_CRANK_SHAFT/1
  DRIVETRAIN_STABILIZATION/2 -> TO_ASM_CLUTCH/1
  DRIVETRAIN_STABILIZATION/3 -> TO_ASM_CENTRAL_DIFFERENTIAL/1
  DRIVETRAIN_STABILIZATION/4 -> TO_ASM_FRONT_DIFFERENTIAL/1
  DRIVETRAIN_STABILIZATION/5 -> TO_ASM_REAR_DIFFERENTIAL/1
  DRIVETRAIN_STABILIZATION/6 -> TO_ASM_CLUTCH_4WD/1
  FROM_ASM_CRANK_SHAFT/1 -> DRIVETRAIN_STABILIZATION/2
  FROM_ASM_CLUTCH/1 -> DRIVETRAIN_STABILIZATION/3
  FROM_ASM_GEARBOX/1 -> DRIVETRAIN_STABILIZATION/4
  FROM_ASM_TORQUE_CONVERTER/1 -> DRIVETRAIN_STABILIZATION/5
  FROM_ASM_CENTRAL_DIFFERENTIAL/1 -> DRIVETRAIN_STABILIZATION/6
  FROM_ASM_SHAFT_CR/1 -> DRIVETRAIN_STABILIZATION/8
  FROM_ASM_REAR_DIFFERENTIAL/1 -> DRIVETRAIN_STABILIZATION/10
  FROM_ASM_TRANSFER_GEARBOX/1 -> DRIVETRAIN_STABILIZATION/16
  FROM_ASM_SHAFT_FR/1 -> DRIVETRAIN_STABILIZATION/12
  FROM_ASM_SHAFT_RR/1 -> DRIVETRAIN_STABILIZATION/14
  FROM_ASM_SHAFT_CF/1 -> DRIVETRAIN_STABILIZATION/7
  FROM_ASM_CLUTCH_4WD/1 -> DRIVETRAIN_STABILIZATION/17
  FROM_ASM_SHAFT_TGCL4WD/1 -> DRIVETRAIN_STABILIZATION/15
  FROM_ASM_SHAFT_RL/1 -> DRIVETRAIN_STABILIZATION/13
  FROM_ASM_SHAFT_FL/1 -> DRIVETRAIN_STABILIZATION/11
  FROM_ASM_FRONT_DIFFERENTIAL/1 -> DRIVETRAIN_STABILIZATION/9

== system ASM_Traffic_V2X_Complete_Model_2/MDL/Drivetrain/Final_Drive_Assembly/Shafts ==
  omega_Out_Right_RearDiff[rad|s] : Inport
  omega_Out_Left_RearDiff[rad|s] : Inport  Port=2
  omega_Out_Right_FrontDiff[rad|s] : Inport  Port=3
  omega_Out_Left_FrontDiff[rad|s] : Inport  Port=4
  omega_Out_Rear_CentralDiff[rad|s] : Inport  Port=5
  omega_Out_Front_CentralDiff[rad|s] : Inport  Port=6
  omega_In_FrontDiff[rad|s] : Inport  Port=7
  omega_In_RearDiff[rad|s] : Inport  Port=8
  omega_Wheel[FL,FR,RL,RR][rad|s] : Inport  Port=9
  Reset[0|1] : Inport  Port=10
  Demux : Demux
  Map_Mode_2_Parameter : Lookup_n-D  NumberOfTableDimensions=1  BreakpointsForDimension1=[1:5]  Table=[1 2 3 1 2]  InternalRulePriority=Speed  RndMeth=Simplest  InputSameDT=on
      settings: AttributesFormatString=Map FF => FWD & FF4WD => AWD
  Mux : Mux
  SHAFT_CF : ASM_VehicleDynamics_lib/Drivetrain/Shaft/SHAFT_CF  Tag=ASM_SUBCOMPONENT  Const_Stiffenss_FourWheelDrive=MDL.Drivetrain.Shaft_CF.FourWheelDrive.Const_Stiffness  Const_Damping_FourWheelDrive=MDL.Drivetrain.Shaft_CF.FourWheelDrive.Const_Damping  Const_Stiffenss_FrontWheelDrive=MDL.Drivetrain.Shaft_CF.FrontWheelDrive.Const_Stiffness  Const_Damping_FrontWheelDrive=MDL.Drivetrain.Shaft_CF.FrontWheelDrive.Const_Damping  StepSize=SIM.StepSize  ASMProperties=struct('Name','SHAFT_CF','Version','6.0','Library','ASM_VehicleDynamics_lib')  ASMInstanceName=Shafts  ASMInstanceID=1
  SHAFT_CR : ASM_VehicleDynamics_lib/Drivetrain/Shaft/SHAFT_CR  Tag=ASM_SUBCOMPONENT  Const_Stiffenss_FourWheelDrive=MDL.Drivetrain.Shaft_CR.FourWheelDrive.Const_Stiffness  Const_Damping_FourWheelDrive=MDL.Drivetrain.Shaft_CR.FourWheelDrive.Const_Damping  Const_Stiffenss_RearWheelDrive=MDL.Drivetrain.Shaft_CR.RearWheelDrive.Const_Stiffness  Const_Damping_RearWheelDrive=MDL.Drivetrain.Shaft_CR.RearWheelDrive.Const_Damping  StepSize=SIM.StepSize  ASMProperties=struct('Name','SHAFT_CR','Version','6.0','Library','ASM_VehicleDynamics_lib')  ASMInstanceName=Shafts  ASMInstanceID=1
  SHAFT_FL : ASM_VehicleDynamics_lib/Drivetrain/Shaft/SHAFT_FL  Tag=ASM_SUBCOMPONENT  Const_Stiffenss_FourWheelDrive=MDL.Drivetrain.Shaft_FL.FourWheelDrive.Const_Stiffness  Const_Damping_FourWheelDrive=MDL.Drivetrain.Shaft_FL.FourWheelDrive.Const_Damping  Const_Stiffenss_FrontWheelDrive=MDL.Drivetrain.Shaft_FL.FrontWheelDrive.Const_Stiffness  Const_Damping_FrontWheelDrive=MDL.Drivetrain.Shaft_FL.FrontWheelDrive.Const_Damping  StepSize=SIM.StepSize  ASMProperties=struct('Name','SHAFT_FL','Version','6.0','Library','ASM_VehicleDynamics_lib')  ASMInstanceName=Shafts  ASMInstanceID=1
  SHAFT_FR : ASM_VehicleDynamics_lib/Drivetrain/Shaft/SHAFT_FR  Tag=ASM_SUBCOMPONENT  Const_Stiffenss_FourWheelDrive=MDL.Drivetrain.Shaft_FR.FourWheelDrive.Const_Stiffness  Const_Damping_FourWheelDrive=MDL.Drivetrain.Shaft_FR.FourWheelDrive.Const_Damping  Const_Stiffenss_FrontWheelDrive=MDL.Drivetrain.Shaft_FR.FrontWheelDrive.Const_Stiffness  Const_Damping_FrontWheelDrive=MDL.Drivetrain.Shaft_FR.FrontWheelDrive.Const_Damping  StepSize=SIM.StepSize  ASMProperties=struct('Name','SHAFT_FR','Version','6.0','Library','ASM_VehicleDynamics_lib')  ASMInstanceName=Shafts  ASMInstanceID=1
  SHAFT_RL : ASM_VehicleDynamics_lib/Drivetrain/Shaft/SHAFT_RL  Tag=ASM_SUBCOMPONENT  Const_Stiffenss_FourWheelDrive=MDL.Drivetrain.Shaft_RL.FourWheelDrive.Const_Stiffness  Const_Damping_FourWheelDrive=MDL.Drivetrain.Shaft_RL.FourWheelDrive.Const_Damping  Const_Stiffenss_RearWheelDrive=MDL.Drivetrain.Shaft_RL.RearWheelDrive.Const_Stiffness  Const_Damping_RearWheelDrive=MDL.Drivetrain.Shaft_RL.RearWheelDrive.Const_Damping  StepSize=SIM.StepSize  ASMProperties=struct('Name','SHAFT_RL','Version','6.0','Library','ASM_VehicleDynamics_lib')  ASMInstanceName=Shafts  ASMInstanceID=1
  SHAFT_RR : ASM_VehicleDynamics_lib/Drivetrain/Shaft/SHAFT_RR  Tag=ASM_SUBCOMPONENT  Const_Stiffenss_FourWheelDrive=MDL.Drivetrain.Shaft_RR.FourWheelDrive.Const_Stiffness  Const_Damping_FourWheelDrive=MDL.Drivetrain.Shaft_RR.FourWheelDrive.Const_Damping  Const_Stiffenss_RearWheelDrive=MDL.Drivetrain.Shaft_RR.RearWheelDrive.Const_Stiffness  Const_Damping_RearWheelDrive=MDL.Drivetrain.Shaft_RR.RearWheelDrive.Const_Damping  StepSize=SIM.StepSize  ASMProperties=struct('Name','SHAFT_RR','Version','6.0','Library','ASM_VehicleDynamics_lib')  ASMInstanceName=Shafts  ASMInstanceID=1
  TO_STABILIZATION_SHAFT_CF : ASM_VehicleDynamics_lib/Drivetrain/Stabilization/TO_STABILIZATION  Tag=ASM_SUBCOMPONENT  Stabi_Block=SHAFT_CF  Stabi_Block_ID=1  ASMProperties=struct('Name','TO_STABILIZATION','Version','1.0','Library','ASM_VehicleDynamics_lib')  ASMInstanceName=to_stabilization  ASMInstanceID=1
      settings: AttributesFormatString=Source: SHAFT_CF_ID1
  TO_STABILIZATION_SHAFT_CR : ASM_VehicleDynamics_lib/Drivetrain/Stabilization/TO_STABILIZATION  Tag=ASM_SUBCOMPONENT  Stabi_Block=SHAFT_CR  Stabi_Block_ID=1  ASMProperties=struct('Name','TO_STABILIZATION','Version','1.0','Library','ASM_VehicleDynamics_lib')  ASMInstanceName=to_stabilization  ASMInstanceID=1
      settings: AttributesFormatString=Source: SHAFT_CR_ID1
  TO_STABILIZATION_SHAFT_FL : ASM_VehicleDynamics_lib/Drivetrain/Stabilization/TO_STABILIZATION  Tag=ASM_SUBCOMPONENT  Stabi_Block=SHAFT_FL  Stabi_Block_ID=1  ASMProperties=struct('Name','TO_STABILIZATION','Version','1.0','Library','ASM_VehicleDynamics_lib')  ASMInstanceName=to_stabilization  ASMInstanceID=1
      settings: AttributesFormatString=Source: SHAFT_FL_ID1
  TO_STABILIZATION_SHAFT_FR : ASM_VehicleDynamics_lib/Drivetrain/Stabilization/TO_STABILIZATION  Tag=ASM_SUBCOMPONENT  Stabi_Block=SHAFT_FR  Stabi_Block_ID=1  ASMProperties=struct('Name','TO_STABILIZATION','Version','1.0','Library','ASM_VehicleDynamics_lib')  ASMInstanceName=to_stabilization  ASMInstanceID=1
      settings: AttributesFormatString=Source: SHAFT_FR_ID1
  TO_STABILIZATION_SHAFT_RL : ASM_VehicleDynamics_lib/Drivetrain/Stabilization/TO_STABILIZATION  Tag=ASM_SUBCOMPONENT  Stabi_Block=SHAFT_RL  Stabi_Block_ID=1  ASMProperties=struct('Name','TO_STABILIZATION','Version','1.0','Library','ASM_VehicleDynamics_lib')  ASMInstanceName=to_stabilization  ASMInstanceID=1
      settings: AttributesFormatString=Source: SHAFT_RL_ID1
  TO_STABILIZATION_SHAFT_RR : ASM_VehicleDynamics_lib/Drivetrain/Stabilization/TO_STABILIZATION  Tag=ASM_SUBCOMPONENT  Stabi_Block=SHAFT_RR  Stabi_Block_ID=1  ASMProperties=struct('Name','TO_STABILIZATION','Version','1.0','Library','ASM_VehicleDynamics_lib')  ASMInstanceName=to_stabilization  ASMInstanceID=1
      settings: AttributesFormatString=Source: SHAFT_RR_ID1
  Trq_FR_Shaft[Nm] : Outport
  Trq_FL_Shaft[Nm] : Outport  Port=2
  Trq_CF_Shaft[Nm] : Outport  Port=3
  Trq_CR_Shaft[Nm] : Outport  Port=4
  Trq_RR_Shaft[Nm] : Outport  Port=5
  Trq_RL_Shaft[Nm] : Outport  Port=6
  Trq_Shaft[FL,FR,RL,RR][Nm] : Outport  Port=7
  tag scope: ASMBUS_Drivetrain_Shaft_CF=scoped, ASMBUS_Drivetrain_Shaft_CR=scoped, ASMBUS_Drivetrain_Shaft_FL=scoped, ASMBUS_Drivetrain_Shaft_FR=scoped, ASMBUS_Drivetrain_Shaft_RL=scoped, ASMBUS_Drivetrain_Shaft_RR=scoped
  wires:
  SHAFT_RR/1 -> [ASMBUS_Drivetrain_Shaft_RR]
  SHAFT_RL/1 -> [ASMBUS_Drivetrain_Shaft_RL]
  SHAFT_FR/1 -> [ASMBUS_Drivetrain_Shaft_FR]
  SHAFT_FL/1 -> [ASMBUS_Drivetrain_Shaft_FL]
  SHAFT_CR/1 -> [ASMBUS_Drivetrain_Shaft_CR]
  SHAFT_CF/1 -> [ASMBUS_Drivetrain_Shaft_CF]
  Reset[0|1]/1 -> SHAFT_CF/4, SHAFT_CR/4, SHAFT_FL/4, SHAFT_FR/4, SHAFT_RR/4, SHAFT_RL/4
  Map_Mode_2_Parameter/1 -> SHAFT_CF/3, SHAFT_CR/3, SHAFT_FL/3, SHAFT_FR/3, SHAFT_RR/3, SHAFT_RL/3
  SHAFT_FL/2 -> Mux/1, Trq_FL_Shaft[Nm]/1
  SHAFT_FR/2 -> Trq_FR_Shaft[Nm]/1, Mux/2
  SHAFT_RL/2 -> Mux/3, Trq_RL_Shaft[Nm]/1
  SHAFT_RR/2 -> Mux/4, Trq_RR_Shaft[Nm]/1
  [TAG_Sw_Drivetrain_Mode] -> Map_Mode_2_Parameter/1
  omega_In_FrontDiff[rad|s]/1 -> SHAFT_CF/2
  omega_In_RearDiff[rad|s]/1 -> SHAFT_CR/2
  omega_Out_Rear_CentralDiff[rad|s]/1 -> SHAFT_CR/1
  omega_Out_Front_CentralDiff[rad|s]/1 -> SHAFT_CF/1
  SHAFT_CR/2 -> Trq_CR_Shaft[Nm]/1
  SHAFT_CF/2 -> Trq_CF_Shaft[Nm]/1
  omega_Wheel[FL,FR,RL,RR][rad|s]/1 -> Demux/1
  Demux/1 -> SHAFT_FL/2
  Demux/2 -> SHAFT_FR/2
  Demux/3 -> SHAFT_RL/2
  Demux/4 -> SHAFT_RR/2
  omega_Out_Right_RearDiff[rad|s]/1 -> SHAFT_RR/1
  omega_Out_Left_RearDiff[rad|s]/1 -> SHAFT_RL/1
  omega_Out_Right_FrontDiff[rad|s]/1 -> SHAFT_FR/1
  omega_Out_Left_FrontDiff[rad|s]/1 -> SHAFT_FL/1
  Mux/1 -> Trq_Shaft[FL,FR,RL,RR][Nm]/1
  SHAFT_FR/3 -> TO_STABILIZATION_SHAFT_FR/1
  SHAFT_RL/3 -> TO_STABILIZATION_SHAFT_RL/1
  SHAFT_RR/3 -> TO_STABILIZATION_SHAFT_RR/1
  SHAFT_FL/3 -> TO_STABILIZATION_SHAFT_FL/1
  SHAFT_CR/3 -> TO_STABILIZATION_SHAFT_CR/1
  SHAFT_CF/3 -> TO_STABILIZATION_SHAFT_CF/1

== system ASM_Traffic_V2X_Complete_Model_2/MDL/Drivetrain/Final_Drive_Assembly/SignalSelection ==
  Inertia_Trm[kgm2] : Inport
  Trq_Out_Trm[Nm] : Inport  Port=2
  Trq_In_TransferGearbox[Nm] : Inport  Port=3
  Inertia_In_TransferGearbox[kgm2] : Inport  Port=4
  Trq_Lock_Clutch4WD[Nm] : Inport  Port=5
  Inertia_Out_Clutch4WD[kgm2] : Inport  Port=6
  Trq_CF_Shaft[Nm] : Inport  Port=7
  Trq_CR_Shaft[Nm] : Inport  Port=8
  AWD : simulink/Logic and Bit Operations/Compare To Constant  relop===  const=1  OutDataTypeStr=boolean
  FWD : simulink/Logic and Bit Operations/Compare To Constant  relop===  const=2  OutDataTypeStr=boolean
  NO_Inertia_Ext_Cage_FrontDiff[kgm2] : Constant  Value=0
  NO_Inertia_External_InputShaft_FrontDiff[kgm2] : Constant  Value=0
  NO_Inertia_External_InputShaft_RearDiff[kgm2] : Constant  Value=0
  No_Trq_Ext_Cage_FrontDiff[Nm] : Constant  Value=0
  OR : Logic  Operator=OR  Inputs=3  AllPortsSameDT=off  OutDataTypeStr=boolean
  RWD : simulink/Logic and Bit Operations/Compare To Constant  relop===  const=3  OutDataTypeStr=boolean
  Saturation[1_5] : Saturate  UpperLimit=5  LowerLimit=1
  Switch{,1..5} (6 alike) : Switch  Criteria=u2 ~= 0
  Trq_In_FrontDiff[Nm] : Outport
  Inertia_External_InputShaft_FrontDiff[kgm2] : Outport  Port=2
  Trq_Ext_Cage_FrontDiff[Nm] : Outport  Port=3
  Inertia_Ext_Cage_FrontDiff[kgm2] : Outport  Port=4
  Trq_In_RearDiff[Nm] : Outport  Port=5
  Inertia_External_InputShaft_RearDiff[kgm2] : Outport  Port=6
  wires:
  [TAG_Sw_Drivetrain_Mode] -> Saturation[1_5]/1
  Saturation[1_5]/1 -> AWD/1, FWD/1, RWD/1
  RWD/1 -> OR/3
  FWD/1 -> OR/2
  AWD/1 -> OR/1
  Trq_CF_Shaft[Nm]/1 -> Switch/1
  OR/1 -> Switch1/2, Switch2/2, Switch3/2, Switch5/2, Switch4/2, Switch/2
  Trq_Out_Trm[Nm]/1 -> Switch/3
  Switch/1 -> Trq_In_FrontDiff[Nm]/1
  Switch1/1 -> Inertia_External_InputShaft_FrontDiff[kgm2]/1
  NO_Inertia_External_InputShaft_FrontDiff[kgm2]/1 -> Switch1/1
  Inertia_Trm[kgm2]/1 -> Switch1/3
  Switch2/1 -> Trq_Ext_Cage_FrontDiff[Nm]/1
  Trq_In_TransferGearbox[Nm]/1 -> Switch2/3
  No_Trq_Ext_Cage_FrontDiff[Nm]/1 -> Switch2/1
  Switch3/1 -> Inertia_Ext_Cage_FrontDiff[kgm2]/1
  Inertia_In_TransferGearbox[kgm2]/1 -> Switch3/3
  NO_Inertia_Ext_Cage_FrontDiff[kgm2]/1 -> Switch3/1
  Switch4/1 -> Trq_In_RearDiff[Nm]/1
  Trq_CR_Shaft[Nm]/1 -> Switch4/1
  Trq_Lock_Clutch4WD[Nm]/1 -> Switch4/3
  Switch5/1 -> Inertia_External_InputShaft_RearDiff[kgm2]/1
  NO_Inertia_External_InputShaft_RearDiff[kgm2]/1 -> Switch5/1
  Inertia_Out_Clutch4WD[kgm2]/1 -> Switch5/3

== system ASM_Traffic_V2X_Complete_Model_2/MDL/Drivetrain/Transmission/ASMSignalCollector ==
  SW_TrmMode[] : Inport
  Gear[] : Inport  Port=2
  ActiveTransmission : Subsystem
  BusCreator : BusCreator  Inputs=3
  tag scope: ASMBUS_Transmission=global
  wires:
  Gear[]/1 -> ActiveTransmission/2(Gear[])
  [ASMBUS_Drivetrain_AutomaticTransmission] -> ActiveTransmission/4(AutomaticTransmission), BusCreator/3
  [ASMBUS_Drivetrain_ManualTransmission] -> ActiveTransmission/3(ManualTransmission), BusCreator/2
  ActiveTransmission/1(ActiveTransmission) -> BusCreator/1
  BusCreator/1 -> [ASMBUS_Transmission]  "Transmission"
  SW_TrmMode[]/1 -> ActiveTransmission/1(SW_TrmMode[])
